simulink model "l_proto8k_12tap"  (R2013a)
settings: Solver=VariableStepDiscrete  SolverMode=SingleTasking  StartTime=0.0  StopTime=1000000  RelTol=1e-3
undefined symbols (not defined in the file): pfb_coeff_gen_calc, sfp
libraries: xbsIndex_r4 x16170, casper_library_delays x104, casper_library_misc x63, casper_library_flow_control x4, xps_library x3, xbsReplacements_r4 x2, simulink x1, casper_library_scopes x1
(part 103 of 167)

== system l_proto8k_12tap/fft_wideband_real1/fft_direct/butterfly1_1/twiddle/coeff_gen/cosin ==
  theta : Inport
  misci : Inport  Port=2
  Constant4 : xbsIndex_r4/Constant  const=0  gui_display_data_type=Fixed-point  arith_type=Unsigned  n_bits=1  bin_pt=0  preci_type=Single  exp_width=8  frac_width=24  explicit_period=on  period=1  equ=P=C  opselect=C  inp2=PCIN>>17  opr=+  inp1=P  carry=CIN  dbl_ovrd=off  block_type=constant
  Constant5 : xbsIndex_r4/Constant  const=0  gui_display_data_type=Fixed-point  arith_type=Unsigned  n_bits=1  bin_pt=0  preci_type=Single  exp_width=8  frac_width=24  explicit_period=on  period=1  equ=P=C  opselect=C  inp2=PCIN>>17  opr=+  inp1=P  carry=CIN  dbl_ovrd=off  block_type=constant
  Delay : xbsIndex_r4/Delay  rst=off  infoeditControl=Selection of Reset will increase slice count due to use of real FFs and instead of SRLs  en=off  latency=bram_latency  dbl_ovrd=off  reg_retiming=on  block_type=delay
  Delay10 : xbsIndex_r4/Delay  rst=off  infoeditControl=Selection of Reset will increase slice count due to use of real FFs and instead of SRLs  en=off  latency=bram_latency  dbl_ovrd=off  reg_retiming=on  block_type=delay
  Delay8 : xbsIndex_r4/Delay  rst=off  infoeditControl=Selection of Reset will increase slice count due to use of real FFs and instead of SRLs  en=off  latency=bram_latency  dbl_ovrd=off  reg_retiming=on  block_type=delay
  ROM : xbsIndex_r4/ROM  depth=2^(12)  initVector=[131072 68706500608 68693131264 68680024064 68666916864 68653809664 68640440320 68627333120 68614225921 68601118721 68587749377 68574642177 68561534977 68548427778 68535058434 68521951234 68508844034 68495474691 68482367491 68469260291 68456153092 68442783748 68429676549 68416569349 68403462150 68390092806 68376985607 68363878407 68350771208 68337401864 68324294665 68311187465 68298080266 68284710922 68271603723 68258496524 68245389324 68232019981 68218912782 68205805583 68192436239 68179329040 68166221841 68153114642 68139745299 68126638100 68113530900 68100423701 68087054358 68073947159 68060839960 68047732761 68034363418 68021256219 68008149020 67995041821 67981672478 67968565279 67955458080 67942350882 67928981539 67915874340 67902767141 67889659942 67876290599 67863183401 67850076202 67836969003 67823599661 67810492462 67797385263 67784278065 67770908722 67757801523 67744694325 67731587126 67718217784 67705110585 67692003387 67678896188 67665526846 67652419647 67639312449 67626205250 67612835908 67599728710 67586621511 67573514313 67560144971 67547037772 67533930574 67520823376 67507716178 67494346835 67481239637 67468132439 67455025241 67441655899 67428548701 67415441502 67402334304 67388964962 67375857764 67362750566 67349643368 67336536170 67323166828 67310059630 67296952432 67283845234 67270475893 67257368695 67244261497 67231154299 67218047101 67204677759 67191570562 67178463364 67165356166 67151986824 67138879627 67125772429 67112665231 67099558034 67086188692 67073081495 67059974297 67046867099 67033759902 67020390560 67007283363 66994176165 66981068968 66967961770 66954592429 66941485232 66928378034 66915270837 66902163640 66888794298 66875687101 66862579904 66849472706 66836365509 66822996168 66809888971 66796781773 66783674576 66770567379 66757460182 66744090841 66730983644 66717876447 66704769250 66691662053 66678292711 66665185514 66652078318 66638971121 66625863924 66612756727 66599387386 66586280189 66573172992 66560065795 66546958598 66533851402 66520482061 66507374864 66494267667 66481160470 66468053274 66454946077 66441576736 66428469540 66415362343 66402255146 66389147950 66376040753 66362933557 66349564216 66336457020 66323349823 66310242627 66297135430 66284028234 66270921037 66257551697 66244444501 66231337304 66218230108 66205122911 66192015715 66178908519 66165539179 66152431982 66139324786 66126217590 66113110394 66100003198 66086896001 66073788805 66060681609 66047312269 66034205073 66021097877 66007990681 65994883485 65981776289 65968669093 65955561897 65942454701 65929085361 65915978165 65902870969 65889763773 65876656577 65863549382 65850442186 65837334990 65824227794 65811120598 65798013403 65784644063 65771536867 65758429672 65745322476 65732215280 65719108085 65706000889 65692893694 65679786498 65666679302 65653572107 65640464911 65627357716 65614250520 65600881181 65587773986 65574666790 65561559595 65548452399 65535345204 65522238009 65509130813 65496023618 65482916423 65469809228 65456702032 65443594837 65430487642 65417380447 65404273252 65391166056 65378058861 65364951666 65351844471 65338737276 65325630081 65312522886 65299415691 65286308496 65273201301 65260094106 65246986911 65233879716 65220772521 65207665327 65194558132 65181450937 65168343742 65155236547 65142129352 65129022158 65115914963 65102807768 65089700574 65076593379 65063486184 65050378990 65037271795 65024164600 65011057406 64997950211 64984843017 64971735822 64958628628 64945521433 64932414239 64919307044 64906199850 64893092655 64879985461 64866878267 64853771072 64840663878 64827556684 64814449489 64801342295 64788497245 64775390050 64762282856 64749175662 64736068468 64722961274 64709854080 64696746885 64683639691 64670532497 64657425303 64644318109 64631210915 64618365865 64605258671 64592151477 64579044283 64565937089 64552829895 64539722701 64526615508 64513508314 64500663264 64487556070 64474448876 64461341682 64448234489 64435127295 64422020101 64408912908 64395805714 64382960664 64369853471 64356746277 ...(+45156 chars)]  distributed_mem=Block RAM  rst=off  init_reg=0  en=off  latency=bram_latency  gui_display_data_type=Fixed-point  arith_type=Unsigned  n_bits=n_bits*2  bin_pt=0  preci_type=Single  exp_width=8  frac_width=24  dbl_ovrd=off  optimize=Speed  use_rpm=on  block_type=sprom
  Terminator : Terminator
  Terminator1 : Terminator
  Terminator4 : Terminator
  add_convert0 : Subsystem
  add_convert1 : Subsystem
  assert : xbsIndex_r4/Assert  assert_type=on  type_source=Explicitly  gui_display_data_type=Fixed-point  arith_type=Unsigned  n_bits=12  bin_pt=0  preci_type=Single  exp_width=8  frac_width=24  assert_rate=off  rate_source=Explicitly  period=1  output_port=on  block_type=assert
  c_to_ri : casper_library_misc/c_to_ri  n_bits=n_bits  bin_pt=bin_pt
  invert0 : Subsystem  mask{n_bits=n_bits, bin_pt=bin_pt, neg_latency=neg_latency, mux_latency=mux_latency}
      mask prompts: n_bits "bit width"; bin_pt "binary point"; neg_latency "negate latency"; mux_latency "mux latency"
  invert1 : Subsystem  mask{n_bits=n_bits, bin_pt=bin_pt, neg_latency=neg_latency, mux_latency=mux_latency}
      mask prompts: n_bits "bit width"; bin_pt "binary point"; neg_latency "negate latency"; mux_latency "mux latency"
  -sin : Outport
  -cos : Outport  Port=2
  misco : Outport  Port=3
  wires:
  theta/1 -> assert/1
  assert/1 -> add_convert0/1(theta), add_convert1/1(theta)
  Constant4/1 -> add_convert0/2(misci)
  add_convert0/3(misco) -> Terminator/1
  misci/1 -> add_convert1/2(misci)
  add_convert1/3(misco) -> Delay/1
  add_convert0/2(add) -> ROM/1
  add_convert1/2(add) -> Terminator4/1
  ROM/1 -> c_to_ri/1
  add_convert1/1(negate) -> Delay8/1
  add_convert0/1(negate) -> Delay10/1
  Delay10/1 -> invert0/1(negate)
  Constant5/1 -> invert0/3(misci)
  c_to_ri/1 -> invert0/2(in)
  Delay8/1 -> invert1/1(negate)
  c_to_ri/2 -> invert1/2(in)
  invert0/2(misco) -> Terminator1/1
  Delay/1 -> invert1/3(misci)
  invert0/1(out) -> -sin/1
  invert1/1(out) -> -cos/1
  invert1/2(misco) -> misco/1
